simulink model "case3"  (R2024b)
settings: Solver=FixedStepAuto  StartTime=0  StopTime=1  FixedStep=1e-7  RelTol=1e-3
values from neighbouring files (symbols this model uses):
  SG_D_1_D = 0.01056    [IEEE9_case_parameters.m]    (also in case1_parameters.m; case2_parameters.m; case3_parameters.m; case4_parameters.m)
  SG_D_1_EnableSaturation = 0    [IEEE9_case_parameters.m]    (also in case1_parameters.m; case2_parameters.m; case3_parameters.m; case4_parameters.m)
  SG_D_1_f0 = 60    [IEEE9_case_parameters.m]    (also in case1_parameters.m; case2_parameters.m; case3_parameters.m; case4_parameters.m)
  SG_D_1_H = 7.5    [IEEE9_case_parameters.m]    (also in case1_parameters.m; case2_parameters.m; case3_parameters.m; case4_parameters.m)
  SG_D_1_K_A = 20    [IEEE9_case_parameters.m]    (also in case1_parameters.m; case2_parameters.m; case3_parameters.m; case4_parameters.m)
  SG_D_1_K_E = 1.000000e+1    (= 10)    [IEEE9_case_parameters.m]    (also in case1_parameters.m; case2_parameters.m; case3_parameters.m; case4_parameters.m)
  SG_D_1_K_F = 2.363    [IEEE9_case_parameters.m]    (also in case1_parameters.m; case2_parameters.m; case3_parameters.m; case4_parameters.m)
  SG_D_1_K_s = 0.5    [IEEE9_case_parameters.m]    (also in case1_parameters.m = 5; case2_parameters.m = 5; case3_parameters.m = 5; case4_parameters.m = 5)
  SG_D_1_R_a = 0.001088    [IEEE9_case_parameters.m]    (also in case1_parameters.m; case2_parameters.m; case3_parameters.m; case4_parameters.m)
  SG_D_1_S_A = 1    [IEEE9_case_parameters.m]    (also in case1_parameters.m; case2_parameters.m; case3_parameters.m; case4_parameters.m)
  SG_D_1_S_B = 0.103    [IEEE9_case_parameters.m]    (also in case1_parameters.m; case2_parameters.m; case3_parameters.m; case4_parameters.m)
  SG_D_1_S_N = 10.659857    [IEEE9_case_parameters.m]    (also in case1_parameters.m; case2_parameters.m; case3_parameters.m; case4_parameters.m)
  SG_D_1_SpeedPara = 200    [IEEE9_case_parameters.m]    (also in case1_parameters.m; case2_parameters.m; case3_parameters.m; case4_parameters.m)
  SG_D_1_T_0 = 0.720173    [IEEE9_case_parameters.m]    (also in case1_parameters.m = 0.755522; case2_parameters.m = 0.808931; case3_parameters.m = 0.869402; case4_parameters.m = 0.729316)
  SG_D_1_T_1 = 0.3    [IEEE9_case_parameters.m]    (also in case1_parameters.m; case2_parameters.m; case3_parameters.m; case4_parameters.m)
  SG_D_1_T_2 = 0.05    [IEEE9_case_parameters.m]    (also in case1_parameters.m; case2_parameters.m; case3_parameters.m; case4_parameters.m)
  SG_D_1_T_3 = 0.02    [IEEE9_case_parameters.m]    (also in case1_parameters.m; case2_parameters.m; case3_parameters.m; case4_parameters.m)
  SG_D_1_T_4 = 0.005    [IEEE9_case_parameters.m]    (also in case1_parameters.m; case2_parameters.m; case3_parameters.m; case4_parameters.m)
  SG_D_1_T_A = 0.02    [IEEE9_case_parameters.m]    (also in case1_parameters.m; case2_parameters.m; case3_parameters.m; case4_parameters.m)
  SG_D_1_T_dd = 8.000000e+0    (= 8)    [IEEE9_case_parameters.m]    (also in case1_parameters.m; case2_parameters.m; case3_parameters.m; case4_parameters.m)
  SG_D_1_T_ddd = 0.04    [IEEE9_case_parameters.m]    (also in case1_parameters.m; case2_parameters.m; case3_parameters.m; case4_parameters.m)
  SG_D_1_T_E = 0.314    [IEEE9_case_parameters.m]    (also in case1_parameters.m; case2_parameters.m; case3_parameters.m; case4_parameters.m)
  SG_D_1_T_F = 0.35    [IEEE9_case_parameters.m]    (also in case1_parameters.m; case2_parameters.m; case3_parameters.m; case4_parameters.m)
  SG_D_1_T_qd = 0.8    [IEEE9_case_parameters.m]    (also in case1_parameters.m; case2_parameters.m; case3_parameters.m; case4_parameters.m)
  SG_D_1_T_qdd = 0.02    [IEEE9_case_parameters.m]    (also in case1_parameters.m; case2_parameters.m; case3_parameters.m; case4_parameters.m)
  SG_D_1_T_speed = 0.1    [IEEE9_case_parameters.m]    (also in case1_parameters.m = 200; case2_parameters.m = 200; case3_parameters.m = 200; case4_parameters.m = 200)
  SG_D_1_T_w = 0.5    [IEEE9_case_parameters.m]    (also in case1_parameters.m; case2_parameters.m; case3_parameters.m; case4_parameters.m)
  SG_D_1_V_ref = 1.990276    [IEEE9_case_parameters.m]    (also in case1_parameters.m = 2.042296; case2_parameters.m = 2.051388; case3_parameters.m = 2.089584; case4_parameters.m = 2.01845)
  SG_D_1_w_ref = 376.991118    [IEEE9_case_parameters.m]    (also in case1_parameters.m; case2_parameters.m; case3_parameters.m; case4_parameters.m)
  SG_D_1_wb = 6.000000e+1    (= 60)    [IEEE9_case_parameters.m]    (also in case1_parameters.m; case2_parameters.m; case3_parameters.m; case4_parameters.m)
  SG_D_1_x_d = 1.9    [IEEE9_case_parameters.m]    (also in case1_parameters.m; case2_parameters.m; case3_parameters.m; case4_parameters.m)
  SG_D_1_x_dd = 0.302    [IEEE9_case_parameters.m]    (also in case1_parameters.m; case2_parameters.m; case3_parameters.m; case4_parameters.m)
  SG_D_1_x_ddd = 0.204    [IEEE9_case_parameters.m]    (also in case1_parameters.m; case2_parameters.m; case3_parameters.m; case4_parameters.m)
  SG_D_1_x_l = 0.05    [IEEE9_case_parameters.m]    (also in case1_parameters.m; case2_parameters.m; case3_parameters.m; case4_parameters.m)
  SG_D_1_x_q = 1.3    [IEEE9_case_parameters.m]    (also in case1_parameters.m; case2_parameters.m; case3_parameters.m; case4_parameters.m)
  SG_D_1_x_qd = 0.5    [IEEE9_case_parameters.m]    (also in case1_parameters.m; case2_parameters.m; case3_parameters.m; case4_parameters.m)
  SG_D_1_x_qdd = 0.3    [IEEE9_case_parameters.m]    (also in case1_parameters.m; case2_parameters.m; case3_parameters.m; case4_parameters.m)
  SG_D_2_D = 0.02    [IEEE9_case_parameters.m]    (also in case1_parameters.m; case2_parameters.m; case3_parameters.m; case4_parameters.m)
  SG_D_2_EnableSaturation = 0    [IEEE9_case_parameters.m]    (also in case1_parameters.m; case2_parameters.m; case3_parameters.m; case4_parameters.m)
  SG_D_2_f0 = 60    [IEEE9_case_parameters.m]    (also in case1_parameters.m; case2_parameters.m; case3_parameters.m; case4_parameters.m)
  SG_D_2_H = 8.000000e+0    (= 8)    [IEEE9_case_parameters.m]    (also in case1_parameters.m; case2_parameters.m; case3_parameters.m; case4_parameters.m)
  SG_D_2_K_A = 20    [IEEE9_case_parameters.m]    (also in case1_parameters.m; case2_parameters.m; case3_parameters.m; case4_parameters.m)
  SG_D_2_K_E = 1.000000e+1    (= 10)    [IEEE9_case_parameters.m]    (also in case1_parameters.m; case2_parameters.m; case3_parameters.m; case4_parameters.m)
  SG_D_2_K_F = 2.363    [IEEE9_case_parameters.m]    (also in case1_parameters.m; case2_parameters.m; case3_parameters.m; case4_parameters.m)
  SG_D_2_K_s = 0.5    [IEEE9_case_parameters.m]    (also in case1_parameters.m = 4; case2_parameters.m = 4; case3_parameters.m = 4; case4_parameters.m = 4)
  SG_D_2_R_a = 0.001088    [IEEE9_case_parameters.m]    (also in case1_parameters.m; case2_parameters.m; case3_parameters.m; case4_parameters.m)
  SG_D_2_S_A = 1    [IEEE9_case_parameters.m]    (also in case1_parameters.m; case2_parameters.m; case3_parameters.m; case4_parameters.m)
  SG_D_2_S_B = 0.103    [IEEE9_case_parameters.m]    (also in case1_parameters.m; case2_parameters.m; case3_parameters.m; case4_parameters.m)
  SG_D_2_S_N = 10.659857    [IEEE9_case_parameters.m]    (also in case1_parameters.m; case2_parameters.m; case3_parameters.m; case4_parameters.m)
  SG_D_2_SpeedPara = 200    [IEEE9_case_parameters.m]    (also in case1_parameters.m; case2_parameters.m; case3_parameters.m; case4_parameters.m)
  SG_D_2_T_0 = 1.632913    [IEEE9_case_parameters.m]    (also in case1_parameters.m = 1.632925; case2_parameters.m = 1.632915; case3_parameters.m = 1.632914; case4_parameters.m = 1.632927)
  SG_D_2_T_1 = 0.2    [IEEE9_case_parameters.m]    (also in case1_parameters.m; case2_parameters.m; case3_parameters.m; case4_parameters.m)
  SG_D_2_T_2 = 0.05    [IEEE9_case_parameters.m]    (also in case1_parameters.m; case2_parameters.m; case3_parameters.m; case4_parameters.m)
  SG_D_2_T_3 = 0.02    [IEEE9_case_parameters.m]    (also in case1_parameters.m; case2_parameters.m; case3_parameters.m; case4_parameters.m)
  SG_D_2_T_4 = 0.005    [IEEE9_case_parameters.m]    (also in case1_parameters.m; case2_parameters.m; case3_parameters.m; case4_parameters.m)
  SG_D_2_T_A = 0.02    [IEEE9_case_parameters.m]    (also in case1_parameters.m; case2_parameters.m; case3_parameters.m; case4_parameters.m)
  SG_D_2_T_dd = 7.9    [IEEE9_case_parameters.m]    (also in case1_parameters.m; case2_parameters.m; case3_parameters.m; case4_parameters.m)
  SG_D_2_T_ddd = 0.04    [IEEE9_case_parameters.m]    (also in case1_parameters.m; case2_parameters.m; case3_parameters.m; case4_parameters.m)
  SG_D_2_T_E = 0.314    [IEEE9_case_parameters.m]    (also in case1_parameters.m; case2_parameters.m; case3_parameters.m; case4_parameters.m)
  SG_D_2_T_F = 0.35    [IEEE9_case_parameters.m]    (also in case1_parameters.m; case2_parameters.m; case3_parameters.m; case4_parameters.m)
  SG_D_2_T_qd = 0.8    [IEEE9_case_parameters.m]    (also in case1_parameters.m; case2_parameters.m; case3_parameters.m; case4_parameters.m)
  SG_D_2_T_qdd = 0.015    [IEEE9_case_parameters.m]    (also in case1_parameters.m; case2_parameters.m; case3_parameters.m; case4_parameters.m)
  SG_D_2_T_speed = 0.1    [IEEE9_case_parameters.m]    (also in case1_parameters.m = 150; case2_parameters.m = 150; case3_parameters.m = 150; case4_parameters.m = 150)
  SG_D_2_T_w = 0.35    [IEEE9_case_parameters.m]    (also in case1_parameters.m; case2_parameters.m; case3_parameters.m; case4_parameters.m)
  SG_D_2_V_ref = 2.58547    [IEEE9_case_parameters.m]    (also in case1_parameters.m = 2.597896; case2_parameters.m = 2.587136; case3_parameters.m = 2.586042; case4_parameters.m = 2.599679)
  SG_D_2_w_ref = 376.991118    [IEEE9_case_parameters.m]    (also in case1_parameters.m; case2_parameters.m; case3_parameters.m; case4_parameters.m)
  SG_D_2_wb = 6.000000e+1    (= 60)    [IEEE9_case_parameters.m]    (also in case1_parameters.m; case2_parameters.m; case3_parameters.m; case4_parameters.m)
  SG_D_2_x_d = 1.8    [IEEE9_case_parameters.m]    (also in case1_parameters.m; case2_parameters.m; case3_parameters.m; case4_parameters.m)
  SG_D_2_x_dd = 0.302    [IEEE9_case_parameters.m]    (also in case1_parameters.m; case2_parameters.m; case3_parameters.m; case4_parameters.m)
  SG_D_2_x_ddd = 0.204    [IEEE9_case_parameters.m]    (also in case1_parameters.m; case2_parameters.m; case3_parameters.m; case4_parameters.m)
  SG_D_2_x_l = 0.05    [IEEE9_case_parameters.m]    (also in case1_parameters.m; case2_parameters.m; case3_parameters.m; case4_parameters.m)
  SG_D_2_x_q = 1.25    [IEEE9_case_parameters.m]    (also in case1_parameters.m; case2_parameters.m; case3_parameters.m; case4_parameters.m)
  SG_D_2_x_qd = 0.5    [IEEE9_case_parameters.m]    (also in case1_parameters.m; case2_parameters.m; case3_parameters.m; case4_parameters.m)
  SG_D_2_x_qdd = 0.3    [IEEE9_case_parameters.m]    (also in case1_parameters.m; case2_parameters.m; case3_parameters.m; case4_parameters.m)
  SG_D_3_D = 0.02    [IEEE9_case_parameters.m]    (also in case1_parameters.m; case2_parameters.m; case3_parameters.m; case4_parameters.m)
  SG_D_3_EnableSaturation = 0    [IEEE9_case_parameters.m]    (also in case1_parameters.m; case2_parameters.m; case3_parameters.m; case4_parameters.m)
  SG_D_3_f0 = 60    [IEEE9_case_parameters.m]    (also in case1_parameters.m; case2_parameters.m; case3_parameters.m; case4_parameters.m)
  SG_D_3_H = 7.7    [IEEE9_case_parameters.m]    (also in case1_parameters.m; case2_parameters.m; case3_parameters.m; case4_parameters.m)
  SG_D_3_K_A = 20    [IEEE9_case_parameters.m]    (also in case1_parameters.m; case2_parameters.m; case3_parameters.m; case4_parameters.m)
  SG_D_3_K_E = 1.000000e+1    (= 10)    [IEEE9_case_parameters.m]    (also in case1_parameters.m; case2_parameters.m; case3_parameters.m; case4_parameters.m)
  SG_D_3_K_F = 2.363    [IEEE9_case_parameters.m]    (also in case1_parameters.m; case2_parameters.m; case3_parameters.m; case4_parameters.m)
  SG_D_3_K_s = 0.2    [IEEE9_case_parameters.m]    (also in case1_parameters.m = 2; case2_parameters.m = 2; case3_parameters.m = 2; case4_parameters.m = 2)
  SG_D_3_R_a = 0.001088    [IEEE9_case_parameters.m]    (also in case1_parameters.m; case2_parameters.m; case3_parameters.m; case4_parameters.m)
  SG_D_3_S_A = 1    [IEEE9_case_parameters.m]    (also in case1_parameters.m; case2_parameters.m; case3_parameters.m; case4_parameters.m)
  SG_D_3_S_B = 0.103    [IEEE9_case_parameters.m]    (also in case1_parameters.m; case2_parameters.m; case3_parameters.m; case4_parameters.m)
  SG_D_3_S_N = 10.659857    [IEEE9_case_parameters.m]    (also in case1_parameters.m; case2_parameters.m; case3_parameters.m; case4_parameters.m)
  SG_D_3_SpeedPara = 200    [IEEE9_case_parameters.m]    (also in case1_parameters.m; case2_parameters.m; case3_parameters.m; case4_parameters.m)
  SG_D_3_T_0 = 0.850788    [IEEE9_case_parameters.m]    (also in case1_parameters.m = 0.850786; case2_parameters.m = 0.850787; case3_parameters.m; case4_parameters.m = 0.850786)
  SG_D_3_T_1 = 0.2    [IEEE9_case_parameters.m]    (also in case1_parameters.m; case2_parameters.m; case3_parameters.m; case4_parameters.m)
  SG_D_3_T_2 = 0.05    [IEEE9_case_parameters.m]    (also in case1_parameters.m; case2_parameters.m; case3_parameters.m; case4_parameters.m)
  SG_D_3_T_3 = 0.02    [IEEE9_case_parameters.m]    (also in case1_parameters.m; case2_parameters.m; case3_parameters.m; case4_parameters.m)
  SG_D_3_T_4 = 0.005    [IEEE9_case_parameters.m]    (also in case1_parameters.m; case2_parameters.m; case3_parameters.m; case4_parameters.m)
  SG_D_3_T_A = 0.02    [IEEE9_case_parameters.m]    (also in case1_parameters.m; case2_parameters.m; case3_parameters.m; case4_parameters.m)
  SG_D_3_T_dd = 8.1    [IEEE9_case_parameters.m]    (also in case1_parameters.m; case2_parameters.m; case3_parameters.m; case4_parameters.m)
  SG_D_3_T_ddd = 0.04    [IEEE9_case_parameters.m]    (also in case1_parameters.m; case2_parameters.m; case3_parameters.m; case4_parameters.m)
  SG_D_3_T_E = 0.314    [IEEE9_case_parameters.m]    (also in case1_parameters.m; case2_parameters.m; case3_parameters.m; case4_parameters.m)
  SG_D_3_T_F = 0.35    [IEEE9_case_parameters.m]    (also in case1_parameters.m; case2_parameters.m; case3_parameters.m; case4_parameters.m)
  SG_D_3_T_qd = 0.8    [IEEE9_case_parameters.m]    (also in case1_parameters.m; case2_parameters.m; case3_parameters.m; case4_parameters.m)
  SG_D_3_T_qdd = 0.015    [IEEE9_case_parameters.m]    (also in case1_parameters.m; case2_parameters.m; case3_parameters.m; case4_parameters.m)
  SG_D_3_T_speed = 0.1    [IEEE9_case_parameters.m]    (also in case1_parameters.m = 180; case2_parameters.m = 180; case3_parameters.m = 180; case4_parameters.m = 180)
  SG_D_3_T_w = 0.4    [IEEE9_case_parameters.m]    (also in case1_parameters.m; case2_parameters.m; case3_parameters.m; case4_parameters.m)
  SG_D_3_V_ref = 1.892727    [IEEE9_case_parameters.m]    (also in case1_parameters.m = 1.906439; case2_parameters.m = 1.895535; case3_parameters.m = 1.892105; case4_parameters.m = 1.906598)
  SG_D_3_w_ref = 376.991118    [IEEE9_case_parameters.m]    (also in case1_parameters.m; case2_parameters.m; case3_parameters.m; case4_parameters.m)
  SG_D_3_wb = 6.000000e+1    (= 60)    [IEEE9_case_parameters.m]    (also in case1_parameters.m; case2_parameters.m; case3_parameters.m; case4_parameters.m)
  SG_D_3_x_d = 1.85    [IEEE9_case_parameters.m]    (also in case1_parameters.m; case2_parameters.m; case3_parameters.m; case4_parameters.m)
  SG_D_3_x_dd = 0.302    [IEEE9_case_parameters.m]    (also in case1_parameters.m; case2_parameters.m; case3_parameters.m; case4_parameters.m)
  SG_D_3_x_ddd = 0.204    [IEEE9_case_parameters.m]    (also in case1_parameters.m; case2_parameters.m; case3_parameters.m; case4_parameters.m)
  SG_D_3_x_l = 0.05    [IEEE9_case_parameters.m]    (also in case1_parameters.m; case2_parameters.m; case3_parameters.m; case4_parameters.m)
  SG_D_3_x_q = 1.2    [IEEE9_case_parameters.m]    (also in case1_parameters.m; case2_parameters.m; case3_parameters.m; case4_parameters.m)
  SG_D_3_x_qd = 0.5    [IEEE9_case_parameters.m]    (also in case1_parameters.m; case2_parameters.m; case3_parameters.m; case4_parameters.m)
  SG_D_3_x_qdd = 0.3    [IEEE9_case_parameters.m]    (also in case1_parameters.m; case2_parameters.m; case3_parameters.m; case4_parameters.m)
(part 11 of 12)

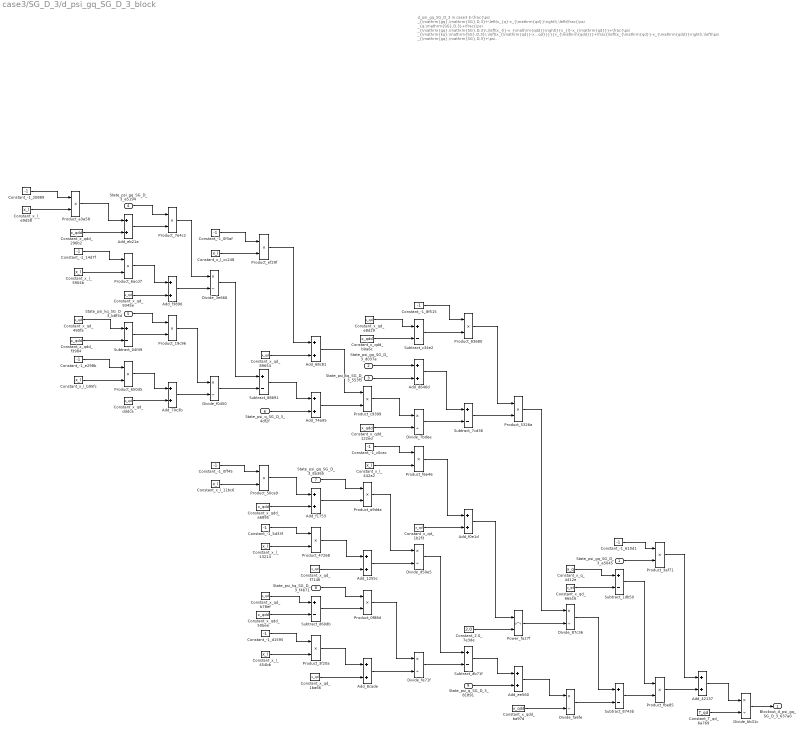
== system case3/SG_D_3/d_psi_gq_SG_D_3_block ==
  note: d_psi_gq_SG_D_3 in case3
      | $-\frac{\psi _{\mathrm{gq},\mathrm{SG},D,3}+\left(x_{q}-x_{\mathrm{qd}}\right)\,\left(\frac{\psi _{q,\mathrm{SG},D,3}+\frac{\psi _{\mathrm{gq},\mathrm{SG},D,3}\,\left(x_{l}-x_{\mathrm{qdd}}\right)}{x_{l}-x_{\mathrm{qd}}}+\frac{\psi _{\mathrm{kq},\mathrm{SG},D,3}\,\left(x_{\mathrm{qd}}-x_{\mathrm{qdd}}\right)}{x_{l}-x_{\mathrm{qd}}}}{x_{\mathrm{qdd}}}+\frac{\left(x_{\mathrm{qd}}-x_{\mathrm{qdd}}\right)\,\left(\psi _{\mathrm{gq},\mathrm{SG},D,3}+\psi _{\mathrm{kq},\mathrm{SG},D,3}+\frac{\left(x_{l}-x_{\mathrm{qd}}\right)\,\left(\psi _{q,\mathrm{SG},D,3}+\frac{\psi _{\mathrm{gq},\mathrm{SG},D,3}\,\left(x_{l}-x_{\mathrm{qdd}}\right)}{x_{l}-x_{\mathrm{qd}}}+\frac{\psi _{\mathrm{kq},\mathrm{SG},D,3}\,\left(x_{\mathrm{qd}}-x_{\mathrm{qdd}}\right)}{x_{l}-x_{\mathrm{qd}}}\right)}{x_{\mathrm{qdd}}}\right)}{{\left(x_{l}-x_{\mathrm{qd}}\right)}^2}\right)}{T_{\mathrm{qd}}}$
      | Automatically generated on 2025-10-31 19:01:05 .
  State_psi_gq_SG_D_3_a5045 : Inport
  State_psi_gq_SG_D_3_d037a : Inport  Port=2
  State_psi_kq_SG_D_3_553f5 : Inport  Port=3
  State_psi_gq_SG_D_3_a5194 : Inport  Port=4
  State_psi_kq_SG_D_3_b8f3d : Inport  Port=5
  State_psi_q_SG_D_3_4df2f : Inport  Port=6
  State_psi_gq_SG_D_3_8a365 : Inport  Port=7
  State_psi_kq_SG_D_3_f4b71 : Inport  Port=8
  State_psi_q_SG_D_3_81891 : Inport  Port=9
  Add_1255c : Sum
  Add_42137 : Sum
  Add_68c81 : Sum
  Add_70c3b : Sum
  Add_74a95 : Sum
  Add_8cade : Sum
  Add_d646d : Sum
  Add_eb21a : Sum
  Add_ee560 : Sum
  Add_f0e1d : Sum
  Add_f1753 : Sum
  Add_f3890 : Sum
  Constant_-1_0f3af : Constant  Value=-1
  Constant_-1_0ff45 : Constant  Value=-1
  Constant_-1_14d7f : Constant  Value=-1
  Constant_-1_20889 : Constant  Value=-1
  Constant_-1_5d33f : Constant  Value=-1
  Constant_-1_610d1 : Constant  Value=-1
  Constant_-1_8f515 : Constant  Value=-1
  Constant_-1_c0cac : Constant  Value=-1
  Constant_-1_d1595 : Constant  Value=-1
  Constant_-1_e298b : Constant  Value=-1
  Constant_2.0_7e3de : Constant  Value=2.0
  Constant_T_qd_6a769 : Constant  Value=T_qd
  Constant_x_l_11bc6 : Constant  Value=x_l
  Constant_x_l_13214 : Constant  Value=x_l
  Constant_x_l_442a2 : Constant  Value=x_l
  Constant_x_l_454bb : Constant  Value=x_l
  Constant_x_l_5904b : Constant  Value=x_l
  Constant_x_l_b95fc : Constant  Value=x_l
  Constant_x_l_cc248 : Constant  Value=x_l
  Constant_x_l_e9d58 : Constant  Value=x_l
  Constant_x_q_4412e : Constant  Value=x_q
  Constant_x_qd_1b2f3 : Constant  Value=x_qd
  Constant_x_qd_1ba66 : Constant  Value=x_qd
  Constant_x_qd_490fa : Constant  Value=x_qd
  Constant_x_qd_66a16 : Constant  Value=x_qd
  Constant_x_qd_89654 : Constant  Value=x_qd
  Constant_x_qd_9345e : Constant  Value=x_qd
  Constant_x_qd_b78ef : Constant  Value=x_qd
  Constant_x_qd_dddca : Constant  Value=x_qd
  Constant_x_qd_e8d29 : Constant  Value=x_qd
  Constant_x_qd_f7146 : Constant  Value=x_qd
  Constant_x_qdd_122ed : Constant  Value=x_qdd
  Constant_x_qdd_296b2 : Constant  Value=x_qdd
  Constant_x_qdd_50bee : Constant  Value=x_qdd
  Constant_x_qdd_a6895 : Constant  Value=x_qdd
  Constant_x_qdd_b0a6c : Constant  Value=x_qdd
  Constant_x_qdd_ba97d : Constant  Value=x_qdd
  Constant_x_qdd_f3984 : Constant  Value=x_qdd
  Divide_3e666 : Product  Inputs=*/
  Divide_7bdee : Product  Inputs=*/
  Divide_87c36 : Product  Inputs=*/
  Divide_bb31c : Product  Inputs=*/
  Divide_d50e5 : Product  Inputs=*/
  Divide_f0450 : Product  Inputs=*/
  Divide_fa6fe : Product  Inputs=*/
  Divide_fe71f : Product  Inputs=*/
  Power_fa27f : Math  Operator=pow
  Product_0f88d : Product
  Product_19c96 : Product
  Product_3af71 : Product
  Product_3f20a : Product
  Product_47268 : Product
  Product_50ca9 : Product
  Product_5326a : Product
  Product_650d5 : Product
  Product_6acd7 : Product
  Product_7e4c2 : Product
  Product_83680 : Product
  Product_a3a58 : Product
  Product_a9dda : Product
  Product_c9399 : Product
  Product_ef29f : Product
  Product_f6e46 : Product
  Product_fbe85 : Product
  Subtract_04f49 : Sum  Inputs=+-
  Subtract_1db50 : Sum  Inputs=+-
  Subtract_7cd36 : Sum  Inputs=+-
  Subtract_8743b : Sum  Inputs=+-
  Subtract_88691 : Sum  Inputs=+-
  Subtract_c34e2 : Sum  Inputs=+-
  Subtract_d60db : Sum  Inputs=+-
  Subtract_db71f : Sum  Inputs=+-
  Blockout_d_psi_gq_SG_D_3_637a0 : Outport
  wires:
  Constant_x_l_442a2/1 -> Product_f6e46/2
  Constant_x_qd_490fa/1 -> Subtract_04f49/1
  Add_68c81/1 -> Product_c9399/1
  Constant_-1_20889/1 -> Product_a3a58/1
  Add_eb21a/1 -> Product_7e4c2/2
  Constant_x_qdd_f3984/1 -> Subtract_04f49/2
  Constant_x_qd_89654/1 -> Add_68c81/2
  Constant_x_l_e9d58/1 -> Product_a3a58/2
  Constant_x_l_5904b/1 -> Product_6acd7/2
  Add_8cade/1 -> Divide_fe71f/2
  State_psi_kq_SG_D_3_553f5/1 -> Add_d646d/2
  Constant_x_qdd_296b2/1 -> Add_eb21a/2
  Product_a3a58/1 -> Add_eb21a/1
  Constant_x_qd_1ba66/1 -> Add_8cade/2
  Product_83680/1 -> Product_5326a/1
  Constant_-1_0ff45/1 -> Product_50ca9/1
  Constant_-1_14d7f/1 -> Product_6acd7/1
  Constant_-1_e298b/1 -> Product_650d5/1
  Constant_x_l_b95fc/1 -> Product_650d5/2
  Constant_-1_8f515/1 -> Product_83680/1
  Constant_-1_610d1/1 -> Product_3af71/1
  State_psi_gq_SG_D_3_a5194/1 -> Product_7e4c2/1
  Product_50ca9/1 -> Add_f1753/1
  Product_6acd7/1 -> Add_f3890/1
  Product_3f20a/1 -> Add_8cade/1
  Constant_x_qd_9345e/1 -> Add_f3890/2
  Constant_-1_5d33f/1 -> Product_47268/1
  State_psi_kq_SG_D_3_b8f3d/1 -> Product_19c96/1
  Subtract_04f49/1 -> Product_19c96/2
  Product_650d5/1 -> Add_70c3b/1
  Add_f1753/1 -> Product_a9dda/2
  Add_f3890/1 -> Divide_3e666/2
  Constant_x_qd_dddca/1 -> Add_70c3b/2
  Product_7e4c2/1 -> Divide_3e666/1
  Constant_T_qd_6a769/1 -> Divide_bb31c/2
  Product_47268/1 -> Add_1255c/1
  Product_19c96/1 -> Divide_f0450/1
  Product_0f88d/1 -> Divide_fe71f/1
  Add_70c3b/1 -> Divide_f0450/2
  Constant_-1_0f3af/1 -> Product_ef29f/1
  Constant_x_qdd_122ed/1 -> Divide_7bdee/2
  Constant_x_l_cc248/1 -> Product_ef29f/2
  Divide_3e666/1 -> Subtract_88691/1
  Constant_x_qd_66a16/1 -> Subtract_1db50/2
  Add_1255c/1 -> Divide_d50e5/2
  Divide_f0450/1 -> Subtract_88691/2
  Constant_x_l_11bc6/1 -> Product_50ca9/2
  Product_ef29f/1 -> Add_68c81/1
  Constant_-1_c0cac/1 -> Product_f6e46/1
  Constant_x_l_13214/1 -> Product_47268/2
  Subtract_88691/1 -> Add_74a95/1
  State_psi_q_SG_D_3_4df2f/1 -> Add_74a95/2
  Constant_-1_d1595/1 -> Product_3f20a/1
  Constant_x_qdd_a6895/1 -> Add_f1753/2
  Constant_x_qd_b78ef/1 -> Subtract_d60db/1
  Constant_x_qdd_50bee/1 -> Subtract_d60db/2
  Constant_x_l_454bb/1 -> Product_3f20a/2
  Add_74a95/1 -> Product_c9399/2
  Constant_x_qdd_b0a6c/1 -> Subtract_c34e2/2
  State_psi_gq_SG_D_3_8a365/1 -> Product_a9dda/1
  Constant_x_qd_f7146/1 -> Add_1255c/2
  Divide_87c36/1 -> Subtract_8743b/1
  State_psi_kq_SG_D_3_f4b71/1 -> Product_0f88d/1
  Subtract_d60db/1 -> Product_0f88d/2
  Constant_x_qd_e8d29/1 -> Subtract_c34e2/1
  State_psi_gq_SG_D_3_d037a/1 -> Add_d646d/1
  Product_c9399/1 -> Divide_7bdee/1
  Product_a9dda/1 -> Divide_d50e5/1
  Subtract_c34e2/1 -> Product_83680/2
  Add_d646d/1 -> Subtract_7cd36/1
  Divide_7bdee/1 -> Subtract_7cd36/2
  Product_f6e46/1 -> Add_f0e1d/1
  Constant_x_qd_1b2f3/1 -> Add_f0e1d/2
  Divide_d50e5/1 -> Subtract_db71f/1
  Divide_fe71f/1 -> Subtract_db71f/2
  Subtract_7cd36/1 -> Product_5326a/2
  Add_f0e1d/1 -> Power_fa27f/1
  Constant_2.0_7e3de/1 -> Power_fa27f/2
  Subtract_db71f/1 -> Add_ee560/1
  State_psi_q_SG_D_3_81891/1 -> Add_ee560/2
  Product_5326a/1 -> Divide_87c36/1
  Power_fa27f/1 -> Divide_87c36/2
  Add_ee560/1 -> Divide_fa6fe/1
  Constant_x_qdd_ba97d/1 -> Divide_fa6fe/2
  Constant_x_q_4412e/1 -> Subtract_1db50/1
  Divide_fa6fe/1 -> Subtract_8743b/2
  State_psi_gq_SG_D_3_a5045/1 -> Product_3af71/2
  Subtract_1db50/1 -> Product_fbe85/1
  Subtract_8743b/1 -> Product_fbe85/2
  Product_3af71/1 -> Add_42137/1
  Product_fbe85/1 -> Add_42137/2
  Add_42137/1 -> Divide_bb31c/1
  Divide_bb31c/1 -> Blockout_d_psi_gq_SG_D_3_637a0/1

== system case3/SG_D_3/d_psi_kq_SG_D_3_block ==
  note: d_psi_kq_SG_D_3 in case3
      | $-\frac{\psi _{\mathrm{gq},\mathrm{SG},D,3}+\psi _{\mathrm{kq},\mathrm{SG},D,3}+\frac{\left(x_{l}-x_{\mathrm{qd}}\right)\,\left(\psi _{q,\mathrm{SG},D,3}+\frac{\psi _{\mathrm{gq},\mathrm{SG},D,3}\,\left(x_{l}-x_{\mathrm{qdd}}\right)}{x_{l}-x_{\mathrm{qd}}}+\frac{\psi _{\mathrm{kq},\mathrm{SG},D,3}\,\left(x_{\mathrm{qd}}-x_{\mathrm{qdd}}\right)}{x_{l}-x_{\mathrm{qd}}}\right)}{x_{\mathrm{qdd}}}}{T_{\mathrm{qdd}}}$
      | Automatically generated on 2025-10-31 19:01:08 .
  State_psi_gq_SG_D_3_080c6 : Inport
  State_psi_kq_SG_D_3_95f78 : Inport  Port=2
  State_psi_gq_SG_D_3_e82df : Inport  Port=3
  State_psi_kq_SG_D_3_7c5b6 : Inport  Port=4
  State_psi_q_SG_D_3_faf2a : Inport  Port=5
  Add_4a1e9 : Sum
  Add_4f0a1 : Sum
  Add_5bbb4 : Sum
  Add_6daa5 : Sum
  Add_ddd0b : Sum
  Add_de31b : Sum
  Constant_-1_51f42 : Constant  Value=-1
  Constant_-1_897e2 : Constant  Value=-1
  Constant_-1_aec43 : Constant  Value=-1
  Constant_-1_d4f6f : Constant  Value=-1
  Constant_-1_f888e : Constant  Value=-1
  Constant_T_qdd_f3401 : Constant  Value=T_qdd
  Constant_x_l_16bf9 : Constant  Value=x_l
  Constant_x_l_22b12 : Constant  Value=x_l
  Constant_x_l_8d77a : Constant  Value=x_l
  Constant_x_l_a1048 : Constant  Value=x_l
  Constant_x_qd_37591 : Constant  Value=x_qd
  Constant_x_qd_8562c : Constant  Value=x_qd
  Constant_x_qd_d563f : Constant  Value=x_qd
  Constant_x_qd_e2037 : Constant  Value=x_qd
  Constant_x_qdd_34e04 : Constant  Value=x_qdd
  Constant_x_qdd_6c634 : Constant  Value=x_qdd
  Constant_x_qdd_a888c : Constant  Value=x_qdd
  Divide_0d164 : Product  Inputs=*/
  Divide_62e2e : Product  Inputs=*/
  Divide_65ecf : Product  Inputs=*/
  Divide_a04ee : Product  Inputs=*/
  Product_04db6 : Product
  Product_0567a : Product
  Product_26c9d : Product
  Product_677ae : Product
  Product_71e1d : Product
  Product_7821e : Product
  Product_bd32b : Product
  Product_e33ee : Product
  Subtract_549c3 : Sum  Inputs=+-
  Subtract_82b3e : Sum  Inputs=+-
  Subtract_f9f0f : Sum  Inputs=+-
  Blockout_d_psi_kq_SG_D_3_45068 : Outport
  wires:
  State_psi_q_SG_D_3_faf2a/1 -> Add_5bbb4/2
  Constant_-1_897e2/1 -> Product_677ae/1
  Constant_-1_f888e/1 -> Product_26c9d/1
  Constant_-1_aec43/1 -> Product_e33ee/1
  Constant_x_l_16bf9/1 -> Product_677ae/2
  Constant_x_qdd_34e04/1 -> Add_4f0a1/2
  Product_7821e/1 -> Add_de31b/1
  Constant_x_l_8d77a/1 -> Product_26c9d/2
  Constant_x_qd_d563f/1 -> Subtract_f9f0f/1
  Product_26c9d/1 -> Add_4f0a1/1
  Constant_x_l_a1048/1 -> Product_bd32b/2
  Constant_x_qdd_a888c/1 -> Subtract_f9f0f/2
  Constant_-1_d4f6f/1 -> Product_7821e/1
  Constant_x_l_22b12/1 -> Product_7821e/2
  State_psi_gq_SG_D_3_e82df/1 -> Product_71e1d/1
  Add_4f0a1/1 -> Product_71e1d/2
  Add_5bbb4/1 -> Product_04db6/2
  Product_677ae/1 -> Add_ddd0b/1
  Constant_x_qd_37591/1 -> Add_ddd0b/2
  State_psi_kq_SG_D_3_7c5b6/1 -> Product_0567a/1
  Subtract_f9f0f/1 -> Product_0567a/2
  Add_ddd0b/1 -> Divide_65ecf/2
  Constant_x_qd_8562c/1 -> Add_de31b/2
  Product_71e1d/1 -> Divide_65ecf/1
  Product_0567a/1 -> Divide_a04ee/1
  Add_de31b/1 -> Divide_a04ee/2
  Constant_-1_51f42/1 -> Product_bd32b/1
  Divide_65ecf/1 -> Subtract_82b3e/1
  Add_4a1e9/1 -> Divide_62e2e/1
  Divide_a04ee/1 -> Subtract_82b3e/2
  Divide_62e2e/1 -> Blockout_d_psi_kq_SG_D_3_45068/1
  Product_bd32b/1 -> Add_6daa5/1
  Constant_x_qd_e2037/1 -> Add_6daa5/2
  Subtract_82b3e/1 -> Add_5bbb4/1
  State_psi_gq_SG_D_3_080c6/1 -> Product_e33ee/2
  Add_6daa5/1 -> Product_04db6/1
  Constant_T_qdd_f3401/1 -> Divide_62e2e/2
  Product_e33ee/1 -> Subtract_549c3/1
  State_psi_kq_SG_D_3_95f78/1 -> Subtract_549c3/2
  Product_04db6/1 -> Divide_0d164/1
  Constant_x_qdd_6c634/1 -> Divide_0d164/2
  Subtract_549c3/1 -> Add_4a1e9/1
  Divide_0d164/1 -> Add_4a1e9/2

== system case3/SG_D_3/d_psi_q_SG_D_3_block ==
  note: d_psi_q_SG_D_3 in case3
      | $2\,\pi \,f_{0}\,\left(v_{d,\mathrm{SG},D,3}\,\cos\left(\theta _{\mathrm{SG},D,3}\right)+v_{q,\mathrm{SG},D,3}\,\sin\left(\theta _{\mathrm{SG},D,3}\right)-\frac{R_{a}\,\left(\psi _{q,\mathrm{SG},D,3}+\frac{\psi _{\mathrm{gq},\mathrm{SG},D,3}\,\left(x_{l}-x_{\mathrm{qdd}}\right)}{x_{l}-x_{\mathrm{qd}}}+\frac{\psi _{\mathrm{kq},\mathrm{SG},D,3}\,\left(x_{\mathrm{qd}}-x_{\mathrm{qdd}}\right)}{x_{l}-x_{\mathrm{qd}}}\right)}{x_{\mathrm{qdd}}}-\frac{\psi _{d,\mathrm{SG},D,3}\,w_{\mathrm{SG},D,3}}{2\,f_{0}\,\pi }\right)$
      | Automatically generated on 2025-10-31 19:00:52 .
  State_psi_gq_SG_D_3_0e7f2 : Inport
  State_psi_kq_SG_D_3_f91e2 : Inport  Port=2
  State_psi_q_SG_D_3_f40ab : Inport  Port=3
  Input_v_d_SG_D_3_58a7d : Inport  Port=4
  State_theta_SG_D_3_99845 : Inport  Port=5
  Input_v_q_SG_D_3_adcaa : Inport  Port=6
  State_theta_SG_D_3_acab9 : Inport  Port=7
  State_psi_d_SG_D_3_d979d : Inport  Port=8
  State_w_SG_D_3_c59e4 : Inport  Port=9
  Add_05c41 : Sum
  Add_7c600 : Sum
  Add_c1e13 : Sum
  Add_e257d : Sum
  Add_e994b : Sum
  Constant_-1_44a68 : Constant  Value=-1
  Constant_-1_8b0e9 : Constant  Value=-1
  Constant_-1_f31e2 : Constant  Value=-1
  Constant_-2.0_7954b : Constant  Value=-2.0
  Constant_2.0_9320b : Constant  Value=2.0
  Constant_R_a_4d491 : Constant  Value=R_a
  Constant_f0_91388 : Constant  Value=f0
  Constant_f0_f59f4 : Constant  Value=f0
  Constant_pi_19894 : Constant  Value=pi
  Constant_pi_61227 : Constant  Value=pi
  Constant_x_l_5befb : Constant  Value=x_l
  Constant_x_l_c481b : Constant  Value=x_l
  Constant_x_l_fcb39 : Constant  Value=x_l
  Constant_x_qd_4725e : Constant  Value=x_qd
  Constant_x_qd_6e71f : Constant  Value=x_qd
  Constant_x_qd_97b9b : Constant  Value=x_qd
  Constant_x_qdd_e8baa : Constant  Value=x_qdd
  Constant_x_qdd_f2a71 : Constant  Value=x_qdd
  Constant_x_qdd_fe972 : Constant  Value=x_qdd
  Divide_15d9c : Product  Inputs=*/
  Divide_3d35e : Product  Inputs=*/
  Divide_54124 : Product  Inputs=*/
  Divide_74135 : Product  Inputs=*/
  MathFunc_cos_65e06 : Trigonometry  Operator=cos
  MathFunc_sin_2f1ab : Trigonometry
  Product_1c82e : Product
  Product_22c4e : Product
  Product_3cb16 : Product
  Product_7e3aa : Product
  Product_813a9 : Product
  Product_81664 : Product
  Product_97b61 : Product
  Product_9c111 : Product
  Product_ae215 : Product
  Product_bd9ab : Product
  Product_ccc5b : Product
  Product_eaa73 : Product
  Product_f09cb : Product
  Product_f8a00 : Product
  Subtract_00be8 : Sum  Inputs=+-
  Subtract_58167 : Sum  Inputs=+-
  Subtract_9b41f : Sum  Inputs=+-
  Subtract_ec433 : Sum  Inputs=+-
  Blockout_d_psi_q_SG_D_3_0df16 : Outport
  wires:
  Constant_x_qd_6e71f/1 -> Subtract_00be8/1
  Constant_pi_61227/1 -> Product_bd9ab/2
  Product_ccc5b/1 -> Divide_54124/1
  Constant_x_l_5befb/1 -> Product_9c111/2
  Constant_f0_f59f4/1 -> Product_22c4e/2
  State_w_SG_D_3_c59e4/1 -> Product_81664/2
  Constant_-1_44a68/1 -> Product_813a9/1
  Constant_x_qdd_f2a71/1 -> Add_c1e13/2
  Input_v_d_SG_D_3_58a7d/1 -> Product_f8a00/1
  Constant_x_qdd_e8baa/1 -> Subtract_00be8/2
  Constant_x_l_fcb39/1 -> Product_813a9/2
  Divide_74135/1 -> Add_7c600/2
  Product_813a9/1 -> Add_c1e13/1
  Constant_2.0_9320b/1 -> Product_bd9ab/1
  Add_05c41/1 -> Product_ccc5b/2
  Constant_-1_8b0e9/1 -> Product_9c111/1
  Constant_x_qd_4725e/1 -> Add_e257d/2
  Constant_-1_f31e2/1 -> Product_f09cb/1
  Subtract_58167/1 -> Subtract_ec433/1
  Constant_x_l_c481b/1 -> Product_f09cb/2
  Subtract_ec433/1 -> Add_7c600/1
  Constant_f0_91388/1 -> Product_7e3aa/2
  State_theta_SG_D_3_acab9/1 -> MathFunc_sin_2f1ab/1
  Constant_x_qd_97b9b/1 -> Add_e994b/2
  State_psi_gq_SG_D_3_0e7f2/1 -> Product_eaa73/1
  Add_c1e13/1 -> Product_eaa73/2
  Product_bd9ab/1 -> Product_7e3aa/1
  Product_9c111/1 -> Add_e994b/1
  State_psi_kq_SG_D_3_f91e2/1 -> Product_1c82e/1
  Subtract_00be8/1 -> Product_1c82e/2
  Product_f09cb/1 -> Add_e257d/1
  MathFunc_sin_2f1ab/1 -> Product_3cb16/2
  Product_eaa73/1 -> Divide_15d9c/1
  Product_7e3aa/1 -> Divide_74135/2
  Add_e994b/1 -> Divide_15d9c/2
  Product_1c82e/1 -> Divide_3d35e/1
  Add_e257d/1 -> Divide_3d35e/2
  Input_v_q_SG_D_3_adcaa/1 -> Product_3cb16/1
  Divide_15d9c/1 -> Subtract_9b41f/1
  Subtract_9b41f/1 -> Add_05c41/1
  Divide_3d35e/1 -> Subtract_9b41f/2
  Divide_54124/1 -> Subtract_58167/1
  State_psi_q_SG_D_3_f40ab/1 -> Add_05c41/2
  Product_3cb16/1 -> Subtract_ec433/2
  Constant_R_a_4d491/1 -> Product_ccc5b/1
  State_theta_SG_D_3_99845/1 -> MathFunc_cos_65e06/1
  Constant_x_qdd_fe972/1 -> Divide_54124/2
  MathFunc_cos_65e06/1 -> Product_f8a00/2
  Constant_-2.0_7954b/1 -> Product_ae215/1
  Product_f8a00/1 -> Subtract_58167/2
  State_psi_d_SG_D_3_d979d/1 -> Product_81664/1
  Constant_pi_19894/1 -> Product_ae215/2
  Product_81664/1 -> Divide_74135/1
  Product_ae215/1 -> Product_22c4e/1
  Product_22c4e/1 -> Product_97b61/1
  Add_7c600/1 -> Product_97b61/2
  Product_97b61/1 -> Blockout_d_psi_q_SG_D_3_0df16/1

== system case3/SG_D_3/d_theta_SG_D_3_block ==
  note: d_theta_SG_D_3 in case3
      | $w_{\mathrm{SG},D,3}-2\,\pi \,f_{0}$
      | Automatically generated on 2025-10-31 19:01:15 .
  State_w_SG_D_3_5b30a : Inport
  Add_d9dc7 : Sum
  Constant_-2.0_5f2d2 : Constant  Value=-2.0
  Constant_f0_d1454 : Constant  Value=f0
  Constant_pi_a4be8 : Constant  Value=pi
  Product_40e5e : Product
  Product_52535 : Product
  Blockout_d_theta_SG_D_3_099ad : Outport
  wires:
  Constant_-2.0_5f2d2/1 -> Product_40e5e/1
  Constant_pi_a4be8/1 -> Product_40e5e/2
  State_w_SG_D_3_5b30a/1 -> Add_d9dc7/2
  Product_40e5e/1 -> Product_52535/1
  Constant_f0_d1454/1 -> Product_52535/2
  Product_52535/1 -> Add_d9dc7/1
  Add_d9dc7/1 -> Blockout_d_theta_SG_D_3_099ad/1

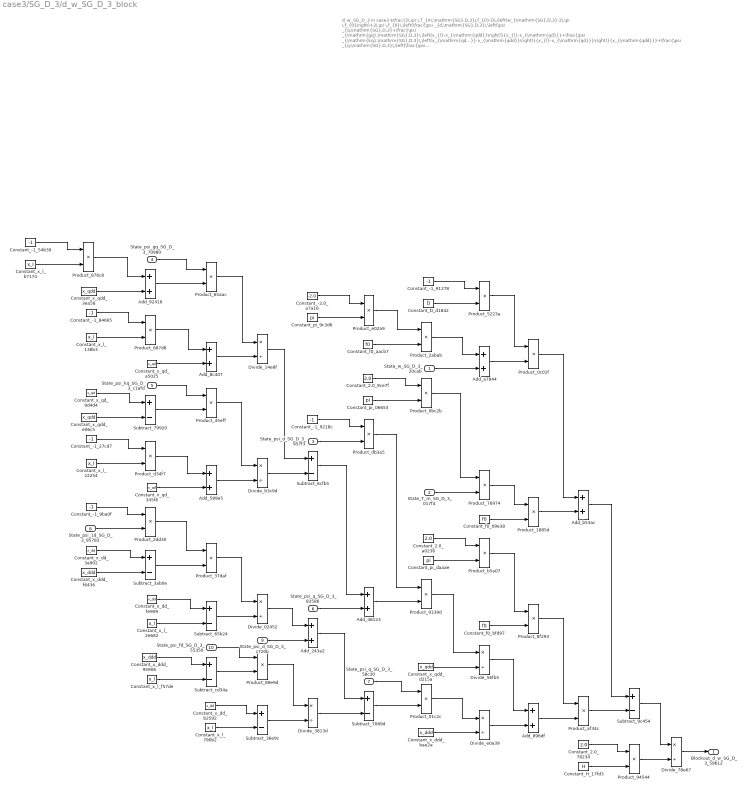
== system case3/SG_D_3/d_w_SG_D_3_block ==
  note: d_w_SG_D_3 in case3
      | $\frac{2\,\pi \,T_{m,\mathrm{SG},D,3}\,f_{0}-D\,\left(w_{\mathrm{SG},D,3}-2\,\pi \,f_{0}\right)+2\,\pi \,f_{0}\,\left(\frac{\psi _{d,\mathrm{SG},D,3}\,\left(\psi _{q,\mathrm{SG},D,3}+\frac{\psi _{\mathrm{gq},\mathrm{SG},D,3}\,\left(x_{l}-x_{\mathrm{qdd}}\right)}{x_{l}-x_{\mathrm{qd}}}+\frac{\psi _{\mathrm{kq},\mathrm{SG},D,3}\,\left(x_{\mathrm{qd}}-x_{\mathrm{qdd}}\right)}{x_{l}-x_{\mathrm{qd}}}\right)}{x_{\mathrm{qdd}}}+\frac{\psi _{q,\mathrm{SG},D,3}\,\left(\frac{\psi _{\mathrm{1d},\mathrm{SG},D,3}\,\left(x_{\mathrm{dd}}-x_{\mathrm{ddd}}\right)}{x_{\mathrm{dd}}-x_{l}}-\psi _{d,\mathrm{SG},D,3}+\frac{\psi _{\mathrm{fd},\mathrm{SG},D,3}\,\left(x_{\mathrm{ddd}}-x_{l}\right)}{x_{\mathrm{dd}}-x_{l}}\right)}{x_{\mathrm{ddd}}}\right)}{2\,H}$
      | Automatically generated on 2025-10-31 19:01:13 .
  State_w_SG_D_3_20cab : Inport
  State_T_m_SG_D_3_017f4 : Inport  Port=2
  State_psi_d_SG_D_3_957f3 : Inport  Port=3
  State_psi_gq_SG_D_3_70980 : Inport  Port=4
  State_psi_kq_SG_D_3_c1afd : Inport  Port=5
  State_psi_q_SG_D_3_83586 : Inport  Port=6
  State_psi_q_SG_D_3_58c30 : Inport  Port=7
  State_psi_1d_SG_D_3_95783 : Inport  Port=8
  State_psi_d_SG_D_3_c720b : Inport  Port=9
  State_psi_fd_SG_D_3_55350 : Inport  Port=10
  Add_243a2 : Sum
  Add_48123 : Sum
  Add_589e5 : Sum
  Add_896df : Sum
  Add_8c407 : Sum
  Add_92416 : Sum
  Add_a7844 : Sum
  Add_b53ac : Sum
  Constant_-1_27cd7 : Constant  Value=-1
  Constant_-1_54b39 : Constant  Value=-1
  Constant_-1_84665 : Constant  Value=-1
  Constant_-1_91278 : Constant  Value=-1
  Constant_-1_9218c : Constant  Value=-1
  Constant_-1_9ba0f : Constant  Value=-1
  Constant_-2.0_a7a16 : Constant  Value=-2.0
  Constant_2.0_78234 : Constant  Value=2.0
  Constant_2.0_9ce7f : Constant  Value=2.0
  Constant_2.0_a0236 : Constant  Value=2.0
  Constant_D_d1842 : Constant  Value=D
  Constant_H_17fd3 : Constant  Value=H
  Constant_f0_09e38 : Constant  Value=f0
  Constant_f0_aacb7 : Constant  Value=f0
  Constant_f0_bfd97 : Constant  Value=f0
  Constant_pi_06653 : Constant  Value=pi
  Constant_pi_9c3d6 : Constant  Value=pi
  Constant_pi_daaae : Constant  Value=pi
  Constant_x_dd_3a902 : Constant  Value=x_dd
  Constant_x_dd_b2592 : Constant  Value=x_dd
  Constant_x_dd_fe909 : Constant  Value=x_dd
  Constant_x_ddd_95906 : Constant  Value=x_ddd
  Constant_x_ddd_bae2a : Constant  Value=x_ddd
  Constant_x_ddd_f6436 : Constant  Value=x_ddd
  Constant_x_l_138b3 : Constant  Value=x_l
  Constant_x_l_22254 : Constant  Value=x_l
  Constant_x_l_2e682 : Constant  Value=x_l
  Constant_x_l_790b2 : Constant  Value=x_l
  Constant_x_l_b7174 : Constant  Value=x_l
  Constant_x_l_f57de : Constant  Value=x_l
  Constant_x_qd_345f8 : Constant  Value=x_qd
  Constant_x_qd_9d4d4 : Constant  Value=x_qd
  Constant_x_qd_a5025 : Constant  Value=x_qd
  Constant_x_qdd_3ea58 : Constant  Value=x_qdd
  Constant_x_qdd_d215a : Constant  Value=x_qdd
  Constant_x_qdd_e06c5 : Constant  Value=x_qdd
  Divide_02452 : Product  Inputs=*/
  Divide_14e8f : Product  Inputs=*/
  Divide_3813d : Product  Inputs=*/
  Divide_56fb5 : Product  Inputs=*/
  Divide_78e67 : Product  Inputs=*/
  Divide_b3c9d : Product  Inputs=*/
  Divide_e0a39 : Product  Inputs=*/
  Product_01c2c : Product
  Product_0bc2b : Product
  Product_0c01f : Product
  Product_1885d : Product
  Product_2abab : Product
  Product_2dd30 : Product
  Product_37daf : Product
  Product_45eff : Product
  Product_5223a : Product
  Product_65aac : Product
  Product_76974 : Product
  Product_876c8 : Product
  Product_887d8 : Product
  Product_89e9d : Product
  Product_8f293 : Product
  Product_9139d : Product
  Product_94544 : Product
  Product_af34c : Product
  Product_b5a07 : Product
  Product_d34f7 : Product
  Product_db3a5 : Product
  Product_e02a9 : Product
  Subtract_36e9c : Sum  Inputs=+-
  Subtract_3ab0e : Sum  Inputs=+-
  Subtract_65b24 : Sum  Inputs=+-
  Subtract_6cfb5 : Sum  Inputs=+-
  Subtract_7089d : Sum  Inputs=+-
  Subtract_79920 : Sum  Inputs=+-
  Subtract_9c454 : Sum  Inputs=+-
  Subtract_cd34a : Sum  Inputs=+-
  Blockout_d_w_SG_D_3_59b12 : Outport
  wires:
  Constant_x_qd_9d4d4/1 -> Subtract_79920/1
  Subtract_3ab0e/1 -> Product_37daf/2
  Subtract_9c454/1 -> Divide_78e67/1
  Constant_-1_54b39/1 -> Product_876c8/1
  Add_92416/1 -> Product_65aac/2
  Constant_x_qdd_e06c5/1 -> Subtract_79920/2
  Subtract_cd34a/1 -> Product_89e9d/2
  Constant_x_l_b7174/1 -> Product_876c8/2
  State_psi_d_SG_D_3_c720b/1 -> Add_243a2/2
  Add_8c407/1 -> Divide_14e8f/2
  Constant_x_dd_fe909/1 -> Subtract_65b24/1
  Constant_x_l_138b3/1 -> Product_887d8/2
  Constant_-1_91278/1 -> Product_5223a/1
  Divide_3813d/1 -> Subtract_7089d/2
  Constant_x_ddd_f6436/1 -> Subtract_3ab0e/2
  Constant_x_qdd_3ea58/1 -> Add_92416/2
  Constant_pi_06653/1 -> Product_0bc2b/2
  Product_876c8/1 -> Add_92416/1
  Constant_-2.0_a7a16/1 -> Product_e02a9/1
  Constant_-1_84665/1 -> Product_887d8/1
  Constant_2.0_a0236/1 -> Product_b5a07/1
  Product_e02a9/1 -> Product_2abab/1
  Constant_-1_27cd7/1 -> Product_d34f7/1
  Subtract_6cfb5/1 -> Add_48123/1
  Constant_x_l_22254/1 -> Product_d34f7/2
  Constant_x_l_f57de/1 -> Subtract_cd34a/2
  Constant_-1_9ba0f/1 -> Product_2dd30/1
  State_psi_1d_SG_D_3_95783/1 -> Product_2dd30/2
  Constant_x_dd_3a902/1 -> Subtract_3ab0e/1
  Product_2dd30/1 -> Product_37daf/1
  State_psi_gq_SG_D_3_70980/1 -> Product_65aac/1
  Constant_x_qd_a5025/1 -> Add_8c407/2
  Product_887d8/1 -> Add_8c407/1
  State_psi_kq_SG_D_3_c1afd/1 -> Product_45eff/1
  Subtract_79920/1 -> Product_45eff/2
  Product_b5a07/1 -> Product_8f293/1
  Product_2abab/1 -> Add_a7844/1
  Product_d34f7/1 -> Add_589e5/1
  State_psi_q_SG_D_3_58c30/1 -> Product_01c2c/1
  Constant_x_qd_345f8/1 -> Add_589e5/2
  Constant_x_l_2e682/1 -> Subtract_65b24/2
  Constant_x_ddd_95906/1 -> Subtract_cd34a/1
  Constant_x_l_790b2/1 -> Subtract_36e9c/2
  Product_65aac/1 -> Divide_14e8f/1
  Product_45eff/1 -> Divide_b3c9d/1
  Add_589e5/1 -> Divide_b3c9d/2
  Product_37daf/1 -> Divide_02452/1
  Subtract_65b24/1 -> Divide_02452/2
  Constant_2.0_9ce7f/1 -> Product_0bc2b/1
  State_psi_fd_SG_D_3_55350/1 -> Product_89e9d/1
  Constant_x_dd_b2592/1 -> Subtract_36e9c/1
  Divide_14e8f/1 -> Subtract_6cfb5/1
  Product_89e9d/1 -> Divide_3813d/1
  Divide_b3c9d/1 -> Subtract_6cfb5/2
  Divide_02452/1 -> Add_243a2/1
  Product_af34c/1 -> Subtract_9c454/2
  Subtract_36e9c/1 -> Divide_3813d/2
  Constant_pi_9c3d6/1 -> Product_e02a9/2
  Constant_pi_daaae/1 -> Product_b5a07/2
  Constant_-1_9218c/1 -> Product_db3a5/1
  State_psi_d_SG_D_3_957f3/1 -> Product_db3a5/2
  State_psi_q_SG_D_3_83586/1 -> Add_48123/2
  Add_243a2/1 -> Subtract_7089d/1
  Constant_f0_aacb7/1 -> Product_2abab/2
  Product_db3a5/1 -> Product_9139d/1
  Add_48123/1 -> Product_9139d/2
  Subtract_7089d/1 -> Product_01c2c/2
  Constant_D_d1842/1 -> Product_5223a/2
  State_w_SG_D_3_20cab/1 -> Add_a7844/2
  Product_0bc2b/1 -> Product_76974/1
  State_T_m_SG_D_3_017f4/1 -> Product_76974/2
  Product_9139d/1 -> Divide_56fb5/1
  Constant_x_qdd_d215a/1 -> Divide_56fb5/2
  Product_01c2c/1 -> Divide_e0a39/1
  Constant_x_ddd_bae2a/1 -> Divide_e0a39/2
  Product_5223a/1 -> Product_0c01f/1
  Add_a7844/1 -> Product_0c01f/2
  Product_76974/1 -> Product_1885d/1
  Constant_f0_09e38/1 -> Product_1885d/2
  Constant_f0_bfd97/1 -> Product_8f293/2
  Divide_56fb5/1 -> Add_896df/1
  Divide_e0a39/1 -> Add_896df/2
  Product_0c01f/1 -> Add_b53ac/1
  Product_1885d/1 -> Add_b53ac/2
  Product_8f293/1 -> Product_af34c/1
  Add_896df/1 -> Product_af34c/2
  Add_b53ac/1 -> Subtract_9c454/1
  Constant_2.0_78234/1 -> Product_94544/1
  Constant_H_17fd3/1 -> Product_94544/2
  Product_94544/1 -> Divide_78e67/2
  Divide_78e67/1 -> Blockout_d_w_SG_D_3_59b12/1

== system case3/SG_D_3/i_d_SG_D_3_block ==
  note: i_d_SG_D_3 in case3
      | $\frac{\sin\left(\theta _{\mathrm{SG},D,3}\right)\,\left(\frac{\psi _{\mathrm{1d},\mathrm{SG},D,3}\,\left(x_{\mathrm{dd}}-x_{\mathrm{ddd}}\right)}{x_{\mathrm{dd}}-x_{l}}-\psi _{d,\mathrm{SG},D,3}+\frac{\psi _{\mathrm{fd},\mathrm{SG},D,3}\,\left(x_{\mathrm{ddd}}-x_{l}\right)}{x_{\mathrm{dd}}-x_{l}}\right)}{x_{\mathrm{ddd}}}-\frac{\cos\left(\theta _{\mathrm{SG},D,3}\right)\,\left(\psi _{q,\mathrm{SG},D,3}+\frac{\psi _{\mathrm{gq},\mathrm{SG},D,3}\,\left(x_{l}-x_{\mathrm{qdd}}\right)}{x_{l}-x_{\mathrm{qd}}}+\frac{\psi _{\mathrm{kq},\mathrm{SG},D,3}\,\left(x_{\mathrm{qd}}-x_{\mathrm{qdd}}\right)}{x_{l}-x_{\mathrm{qd}}}\right)}{x_{\mathrm{qdd}}}$
      | Automatically generated on 2025-10-31 19:01:34 .
  State_psi_gq_SG_D_3_b8fc9 : Inport
  State_psi_kq_SG_D_3_ab859 : Inport  Port=2
  State_psi_q_SG_D_3_5bb1f : Inport  Port=3
  State_theta_SG_D_3_64bc2 : Inport  Port=4
  State_psi_1d_SG_D_3_c5249 : Inport  Port=5
  State_psi_d_SG_D_3_e794c : Inport  Port=6
  State_psi_fd_SG_D_3_7ea81 : Inport  Port=7
  State_theta_SG_D_3_abf6f : Inport  Port=8
  Add_09e5a : Sum
  Add_0c7fc : Sum
  Add_906cf : Sum
  Add_99071 : Sum
  Add_e4657 : Sum
  Constant_-1_192cb : Constant  Value=-1
  Constant_-1_25a00 : Constant  Value=-1
  Constant_-1_27207 : Constant  Value=-1
  Constant_-1_7d985 : Constant  Value=-1
  Constant_-1_9b5bf : Constant  Value=-1
  Constant_x_dd_3fb10 : Constant  Value=x_dd
  Constant_x_dd_6b2c8 : Constant  Value=x_dd
  Constant_x_dd_78dd5 : Constant  Value=x_dd
  Constant_x_ddd_3ceb3 : Constant  Value=x_ddd
  Constant_x_ddd_8cf82 : Constant  Value=x_ddd
  Constant_x_ddd_b31ed : Constant  Value=x_ddd
  Constant_x_l_03cc8 : Constant  Value=x_l
  Constant_x_l_07466 : Constant  Value=x_l
  Constant_x_l_23cf7 : Constant  Value=x_l
  Constant_x_l_3f69e : Constant  Value=x_l
  Constant_x_l_9a52b : Constant  Value=x_l
  Constant_x_l_b11e9 : Constant  Value=x_l
  Constant_x_qd_77dad : Constant  Value=x_qd
  Constant_x_qd_7caec : Constant  Value=x_qd
  Constant_x_qd_c2aea : Constant  Value=x_qd
  Constant_x_qdd_11bde : Constant  Value=x_qdd
  Constant_x_qdd_70d43 : Constant  Value=x_qdd
  Constant_x_qdd_d629c : Constant  Value=x_qdd
  Divide_29773 : Product  Inputs=*/
  Divide_2c400 : Product  Inputs=*/
  Divide_58a5f : Product  Inputs=*/
  Divide_5a57b : Product  Inputs=*/
  Divide_c7680 : Product  Inputs=*/
  Divide_db16a : Product  Inputs=*/
  MathFunc_cos_d4342 : Trigonometry  Operator=cos
  MathFunc_sin_d5766 : Trigonometry
  Product_274f4 : Product
  Product_36b8d : Product
  Product_4f714 : Product
  Product_6c7ef : Product
  Product_6ef91 : Product
  Product_7667d : Product
  Product_bd4cc : Product
  Product_c4f7e : Product
  Product_d0251 : Product
  Product_f43ab : Product
  Product_f561f : Product
  Subtract_0a043 : Sum  Inputs=+-
  Subtract_0b4ae : Sum  Inputs=+-
  Subtract_5a561 : Sum  Inputs=+-
  Subtract_70d31 : Sum  Inputs=+-
  Subtract_7ee58 : Sum  Inputs=+-
  Subtract_8a5bf : Sum  Inputs=+-
  Subtract_e3c8e : Sum  Inputs=+-
  Subtract_fefe0 : Sum  Inputs=+-
  Blockout_i_d_SG_D_3_ca1dd : Outport
  wires:
  Constant_x_qd_77dad/1 -> Subtract_e3c8e/1
  Subtract_70d31/1 -> Blockout_i_d_SG_D_3_ca1dd/1
  Constant_-1_27207/1 -> Product_4f714/1
  Constant_x_l_9a52b/1 -> Product_f43ab/2
  Constant_x_qdd_d629c/1 -> Add_906cf/2
  Constant_x_qdd_11bde/1 -> Subtract_e3c8e/2
  Constant_x_l_3f69e/1 -> Product_4f714/2
  Divide_5a57b/1 -> Subtract_70d31/1
  Product_4f714/1 -> Add_906cf/1
  Constant_x_ddd_8cf82/1 -> Subtract_0b4ae/2
  Constant_-1_9b5bf/1 -> Product_f43ab/1
  Constant_-1_7d985/1 -> Product_274f4/1
  Constant_x_l_b11e9/1 -> Product_274f4/2
  State_psi_1d_SG_D_3_c5249/1 -> Product_f561f/2
  State_psi_gq_SG_D_3_b8fc9/1 -> Product_d0251/1
  Product_f561f/1 -> Product_6c7ef/1
  Add_906cf/1 -> Product_d0251/2
  Product_f43ab/1 -> Add_09e5a/1
  Constant_x_qd_c2aea/1 -> Add_09e5a/2
  State_psi_kq_SG_D_3_ab859/1 -> Product_36b8d/1
  Subtract_5a561/1 -> Divide_db16a/2
  Subtract_e3c8e/1 -> Product_36b8d/2
  Product_274f4/1 -> Add_0c7fc/1
  Constant_x_ddd_b31ed/1 -> Subtract_0a043/1
  Constant_x_qd_7caec/1 -> Add_0c7fc/2
  Constant_-1_192cb/1 -> Product_f561f/1
  Constant_x_dd_6b2c8/1 -> Subtract_0b4ae/1
  Product_d0251/1 -> Divide_c7680/1
  Add_09e5a/1 -> Divide_c7680/2
  Product_36b8d/1 -> Divide_2c400/1
  Add_0c7fc/1 -> Divide_2c400/2
  Divide_db16a/1 -> Subtract_7ee58/2
  Subtract_0b4ae/1 -> Product_6c7ef/2
  State_theta_SG_D_3_64bc2/1 -> MathFunc_cos_d4342/1
  Constant_x_dd_3fb10/1 -> Subtract_fefe0/1
  Product_bd4cc/1 -> Product_6ef91/1
  Constant_x_l_07466/1 -> Subtract_fefe0/2
  Add_e4657/1 -> Subtract_7ee58/1
  Constant_x_l_03cc8/1 -> Subtract_0a043/2
  State_theta_SG_D_3_abf6f/1 -> MathFunc_sin_d5766/1
  Divide_c7680/1 -> Subtract_8a5bf/1
  Add_99071/1 -> Product_bd4cc/2
  Divide_2c400/1 -> Subtract_8a5bf/2
  Product_6c7ef/1 -> Divide_29773/1
  Subtract_fefe0/1 -> Divide_29773/2
  State_psi_fd_SG_D_3_7ea81/1 -> Product_c4f7e/1
  Divide_58a5f/1 -> Subtract_70d31/2
  Subtract_0a043/1 -> Product_c4f7e/2
  Constant_x_dd_78dd5/1 -> Subtract_5a561/1
  Subtract_8a5bf/1 -> Add_99071/1
  Constant_x_l_23cf7/1 -> Subtract_5a561/2
  Constant_-1_25a00/1 -> Product_bd4cc/1
  State_psi_q_SG_D_3_5bb1f/1 -> Add_99071/2
  Divide_29773/1 -> Add_e4657/1
  State_psi_d_SG_D_3_e794c/1 -> Add_e4657/2
  Product_c4f7e/1 -> Divide_db16a/1
  MathFunc_cos_d4342/1 -> Product_6ef91/2
  MathFunc_sin_d5766/1 -> Product_7667d/2
  Subtract_7ee58/1 -> Product_7667d/1
  Product_6ef91/1 -> Divide_5a57b/1
  Constant_x_qdd_70d43/1 -> Divide_5a57b/2
  Product_7667d/1 -> Divide_58a5f/1
  Constant_x_ddd_3ceb3/1 -> Divide_58a5f/2
